simulink model "SWC_TCF"  (R2020a)
settings: Solver=FixedStepDiscrete  StartTime=0.0  StopTime=0.01  FixedStep=0.001  RelTol=1e-3
values from neighbouring files (symbols this model uses):
  CAL_TCF_AgTrqTubeCAy_af32 = 0.0    [SWC_TCF_DataDictionary.sldd]
  CAL_TCF_flgUsePlossCompa_b = 0.0    [SWC_TCF_DataDictionary.sldd]
  CAL_TCF_HiSpdDirStop_f32 = 0.0    [SWC_TCF_DataDictionary.sldd]
  CAL_TCF_HiTrqDirStop_f32 = 0.0    [SWC_TCF_DataDictionary.sldd]
  CAL_TCF_IsCutOffFrq_f32 = 0.0    [SWC_TCF_DataDictionary.sldd]
  CAL_TCF_IsPwrLosCAx_af32 = 0.0    [SWC_TCF_DataDictionary.sldd]
  CAL_TCF_LdSubLqCAzGen_af32 = 0.0    [SWC_TCF_DataDictionary.sldd]
  CAL_TCF_LdSubLqCAzMot_af32 = 0.0    [SWC_TCF_DataDictionary.sldd]
  CAL_TCF_LdSubLqIdCAx_af32 = 0.0    [SWC_TCF_DataDictionary.sldd]
  CAL_TCF_LdSubLqIqCAy_af32 = 0.0    [SWC_TCF_DataDictionary.sldd]
  CAL_TCF_LoSpdDirStop_f32 = 0.0    [SWC_TCF_DataDictionary.sldd]
  CAL_TCF_LoTrqDirStop_f32 = 0.0    [SWC_TCF_DataDictionary.sldd]
  CAL_TCF_MotorPole_u8 = 0.0    [SWC_TCF_DataDictionary.sldd]
  CAL_TCF_NPwrLosCAy_af32 = 0.0    [SWC_TCF_DataDictionary.sldd]
  CAL_TCF_Psi_f32 = 0.0    [SWC_TCF_DataDictionary.sldd]
  CAL_TCF_PwrCompaElectCAz_af32 = 0.0    [SWC_TCF_DataDictionary.sldd]
  CAL_TCF_PwrCompaIsCAy_af32 = 0.0    [SWC_TCF_DataDictionary.sldd]
  CAL_TCF_PwrCompaSpdCAx_af32 = 0.0    [SWC_TCF_DataDictionary.sldd]
  CAL_TCF_PwrInputCutOffFrq_f32 = 0.0    [SWC_TCF_DataDictionary.sldd]
  CAL_TCF_PwrLossCAz_af32 = 0.0    [SWC_TCF_DataDictionary.sldd]
  CAL_TCF_PwrTrqCalcSpdThrH_f32 = 0.0    [SWC_TCF_DataDictionary.sldd]
  CAL_TCF_PwrTrqCalcSpdThrL_f32 = 0.0    [SWC_TCF_DataDictionary.sldd]
  CAL_TCF_PwrTrqTubeCAy_af32 = 0.0    [SWC_TCF_DataDictionary.sldd]
  CAL_TCF_SpeedCtlMode_u8 = 0.0    [SWC_TCF_DataDictionary.sldd]
  CAL_TCF_TempStrMax_f32 = 0.0    [SWC_TCF_DataDictionary.sldd]
  CAL_TCF_TempStrMin_f32 = 0.0    [SWC_TCF_DataDictionary.sldd]
  CAL_TCF_TempStrPlossFact_f32 = 0.0    [SWC_TCF_DataDictionary.sldd]
  CAL_TCF_TrqCalcMonCountTrh_s16 = 0.0    [SWC_TCF_DataDictionary.sldd]
  CAL_TCF_TrqCalcMonDebTrh_s16 = 0.0    [SWC_TCF_DataDictionary.sldd]
  CAL_TCF_TrqCalcMonErrRst_b = 0.0    [SWC_TCF_DataDictionary.sldd]
  CAL_TCF_TrqMechCutOffFrq_f32 = 0.0    [SWC_TCF_DataDictionary.sldd]
  CAL_TCF_TrqTubeNCAx_af32 = 0.0    [SWC_TCF_DataDictionary.sldd]
  GLB_TCF_BwELect_u8 = 0.0    [SWC_TCF_DataDictionary.sldd]
  GLB_TCF_BwGene_u8 = 0.0    [SWC_TCF_DataDictionary.sldd]
  GLB_TCF_CircAge_f32 = 0.0    [SWC_TCF_DataDictionary.sldd]
  GLB_TCF_DigtValue_u16 = 0.0    [SWC_TCF_DataDictionary.sldd]
  GLB_TCF_FwELect_u8 = 0.0    [SWC_TCF_DataDictionary.sldd]
  GLB_TCF_FwGene_u8 = 0.0    [SWC_TCF_DataDictionary.sldd]
  GLB_TCF_MotorBw_u8 = 0.0    [SWC_TCF_DataDictionary.sldd]
  GLB_TCF_MotorFw_u8 = 0.0    [SWC_TCF_DataDictionary.sldd]
  GLB_TCF_MotorStop_u8 = 0.0    [SWC_TCF_DataDictionary.sldd]
  GLB_TCF_NegvTrq_u8 = 0.0    [SWC_TCF_DataDictionary.sldd]
  GLB_TCF_PosvTrq_u8 = 0.0    [SWC_TCF_DataDictionary.sldd]
  GLB_TCF_ZeroTrq_u8 = 0.0    [SWC_TCF_DataDictionary.sldd]
  PRV_CalFltFrq_1ms = 0.0    [SWC_TCF_DataDictionary.sldd]
  PRV_IsCalFltFrq_1ms = 0.0    [SWC_TCF_DataDictionary.sldd]
  Tbl_cos_table = 0.0    [SWC_TCF_DataDictionary.sldd]
  Tbl_sin_table = 0.0    [SWC_TCF_DataDictionary.sldd]
  TCF_PwrCompaGenCAz_af32 = 0.0    [SWC_TCF_DataDictionary.sldd]
undefined symbols (not defined in the file or in its folder): CAL_TOM_AgTrqFltTs_f32, CAL_TOM_PwrTrqFltTs_f32
libraries: simulink x9
(part 2 of 2)

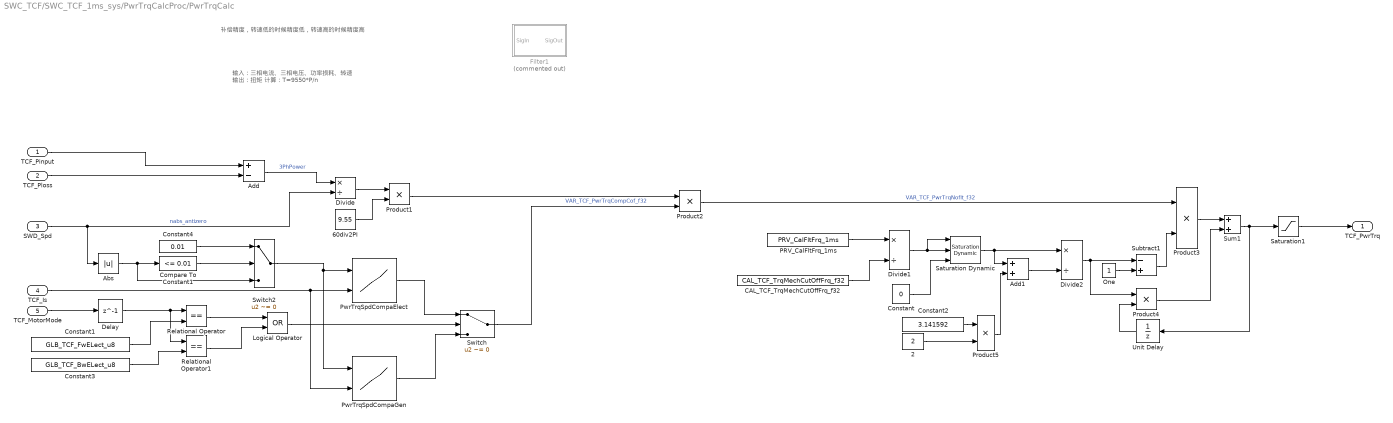
== system SWC_TCF/SWC_TCF_1ms_sys/PwrTrqCalcProc/PwrTrqCalc ==
  note: 补偿精度，转速低的时候精度低，转速高的时候精度高
  note: 输入：三相电流、三相电压、功率损耗、转速
      | 输出：扭矩
      | 计算：T=9550*P/n
  TCF_Pinput : Inport
  TCF_Ploss : Inport  Port=2
  SWD_Spd : Inport  Port=3
  TCF_Is : Inport  Port=4
  TCF_MotorMode : Inport  Port=5
  2 : Constant  Value=2  OutDataTypeStr=single
  60div2PI : Constant  Value=9.55  OutDataTypeStr=single
  Abs : Abs
  Add : Sum  Inputs=+-
  Add1 : Sum
  CAL_TCF_TrqMechCutOffFrq_f32 : Constant  Value=CAL_TCF_TrqMechCutOffFrq_f32
  Compare To Constant1 : simulink/Logic and Bit Operations/Compare To Constant  relop=<=  const=0.01  OutDataTypeStr=boolean
  Constant : Constant  Value=0  OutDataTypeStr=single
  Constant1 : Constant  Value=GLB_TCF_FwELect_u8  OutDataTypeStr=uint8
  Constant2 : Constant  Value=3.141592  OutDataTypeStr=single
  Constant3 : Constant  Value=GLB_TCF_BwELect_u8  OutDataTypeStr=uint8
  Constant4 : Constant  Value=0.01  OutDataTypeStr=single
  Delay : Delay  DelayLength=1  InitialCondition=0
  Divide : Product  Inputs=*/
  Divide1 : Product  Inputs=*/
  Divide2 : Product  Inputs=*/
  Filter1 : Subsystem  Commented=on
  Logical Operator : Logic  Operator=OR  AllPortsSameDT=off  OutDataTypeStr=boolean
  One : Constant  OutDataTypeStr=single
  PRV_CalFltFrq_1ms : Constant  Value=PRV_CalFltFrq_1ms
  Product{1..5} (5 alike) : Product
  PwrTrqSpdCompaElect : Lookup_n-D  BreakpointsForDimension1=CAL_TCF_PwrCompaSpdCAx_af32  BreakpointsForDimension2=CAL_TCF_PwrCompaIsCAy_af32  Table=CAL_TCF_PwrCompaElectCAz_af32  UseLastTableValue=on  InternalRulePriority=Speed  RndMeth=Simplest  InputSameDT=on
  PwrTrqSpdCompaGen : Lookup_n-D  BreakpointsForDimension1=CAL_TCF_PwrCompaSpdCAx_af32  BreakpointsForDimension2=CAL_TCF_PwrCompaIsCAy_af32  Table=TCF_PwrCompaGenCAz_af32  UseLastTableValue=on  InternalRulePriority=Speed  RndMeth=Simplest  InputSameDT=on
  Relational Operator : RelationalOperator  Operator===  OutDataTypeStr=boolean  RndMeth=Simplest
  Relational Operator1 : RelationalOperator  Operator===  OutDataTypeStr=boolean  RndMeth=Simplest
  Saturation Dynamic : simulink/Discontinuities/Saturation Dynamic  OutMin=[]  OutMax=[]  OutDataTypeStr=Inherit: Same as second input  OutDataType=fixdt(1, 16)  OutScaling=2^-10  DoSatur=off
  Saturation1 : Saturate  UpperLimit=500  LowerLimit=-500
  Subtract1 : Sum  Inputs=-+
  Sum1 : Sum
  Switch : Switch  Criteria=u2 ~= 0
  Switch2 : Switch  Criteria=u2 ~= 0
  Unit Delay : UnitDelay  SampleTime=-1  HasFrameUpgradeWarning=on
  TCF_PwrTrq : Outport  VectorParamsAs1DForOutWhenUnconnected=off
  wires:
  SWD_Spd/1 -> Abs/1, Divide/2  "nabs_antizero"
  60div2PI/1 -> Product1/2
  Divide/1 -> Product1/1
  Add/1 -> Divide/1  "3PhPower"
  TCF_Ploss/1 -> Add/2
  Product1/1 -> Product2/1
  TCF_Pinput/1 -> Add/1
  Sum1/1 -> Saturation1/1, Unit Delay/1
  Divide1/1 -> Saturation Dynamic/1, Saturation Dynamic/2
  Product5/1 -> Add1/2
  Product4/1 -> Sum1/2
  Unit Delay/1 -> Product4/2
  One/1 -> Subtract1/2
  Product2/1 -> Product3/1  "VAR_TCF_PwrTrqNoflt_f32"
  Add1/1 -> Divide2/2
  Divide2/1 -> Product4/1, Subtract1/1
  Constant/1 -> Saturation Dynamic/3
  Subtract1/1 -> Product3/2
  PRV_CalFltFrq_1ms/1 -> Divide1/1
  Saturation Dynamic/1 -> Divide2/1, Add1/1
  Product3/1 -> Sum1/1
  2/1 -> Product5/2
  Constant2/1 -> Product5/1
  CAL_TCF_TrqMechCutOffFrq_f32/1 -> Divide1/2
  Saturation1/1 -> TCF_PwrTrq/1
  Switch2/1 -> PwrTrqSpdCompaGen/1, PwrTrqSpdCompaElect/1
  TCF_Is/1 -> PwrTrqSpdCompaGen/2, PwrTrqSpdCompaElect/2
  PwrTrqSpdCompaElect/1 -> Switch/1
  PwrTrqSpdCompaGen/1 -> Switch/3
  TCF_MotorMode/1 -> Delay/1
  Constant3/1 -> Relational Operator1/2
  Relational Operator/1 -> Logical Operator/1
  Constant1/1 -> Relational Operator/2
  Relational Operator1/1 -> Logical Operator/2
  Logical Operator/1 -> Switch/2
  Switch/1 -> Product2/2  "VAR_TCF_PwrTrqCompCof_f32"
  Abs/1 -> Switch2/3, Compare To Constant1/1
  Constant4/1 -> Switch2/1
  Compare To Constant1/1 -> Switch2/2
  Delay/1 -> Relational Operator1/1, Relational Operator/1

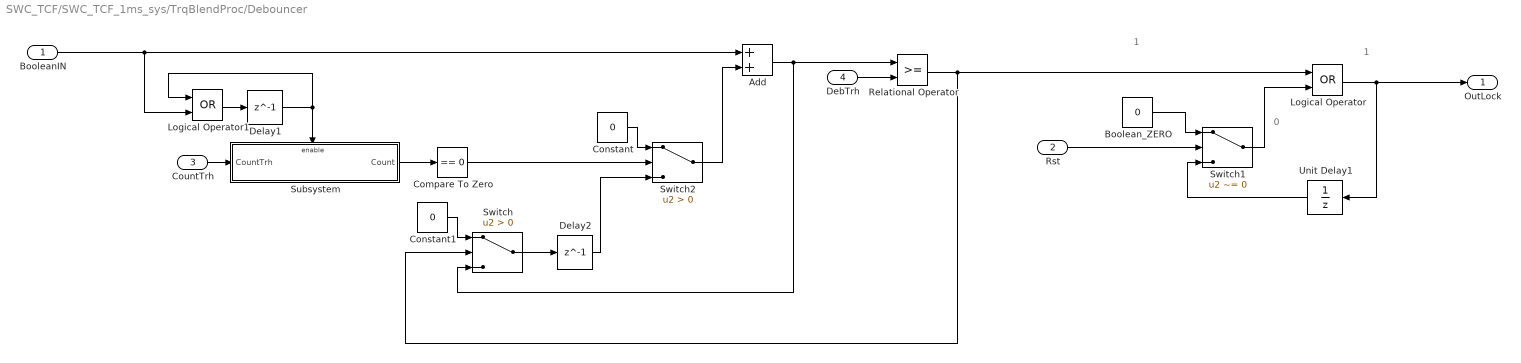
== system SWC_TCF/SWC_TCF_1ms_sys/TrqBlendProc/Debouncer ==
  note: 0
  note: 1
  note: 1
  BooleanIN : Inport
  Rst : Inport  Port=2
  CountTrh : Inport  Port=3
  DebTrh : Inport  Port=4
  Add : Sum
  Boolean_ZERO : Constant  Value=0  OutDataTypeStr=boolean
  Compare To Zero : simulink/Logic and Bit Operations/Compare To Zero  relop===  OutDataTypeStr=boolean
  Constant : Constant  Value=0  OutDataTypeStr=int16
  Constant1 : Constant  Value=0  OutDataTypeStr=int16
  Delay1 : Delay  DelayLength=1
  Delay2 : Delay  DelayLength=1
  Logical Operator : Logic  Operator=OR  AllPortsSameDT=off  OutDataTypeStr=boolean
  Logical Operator1 : Logic  Operator=OR  AllPortsSameDT=off  OutDataTypeStr=boolean
  Relational Operator : RelationalOperator  OutDataTypeStr=boolean  RndMeth=Simplest
  Subsystem : Subsystem
  Switch : Switch  Criteria=u2 > Threshold
  Switch1 : Switch  Criteria=u2 ~= 0
  Switch2 : Switch  Criteria=u2 > Threshold
  Unit Delay1 : UnitDelay  SampleTime=-1  HasFrameUpgradeWarning=on
  OutLock : Outport  VectorParamsAs1DForOutWhenUnconnected=off
  wires:
  Constant1/1 -> Switch/1
  Switch/1 -> Delay2/1
  DebTrh/1 -> Relational Operator/2
  Relational Operator/1 -> Logical Operator/1, Switch/2
  BooleanIN/1 -> Add/1, Logical Operator1/2
  Unit Delay1/1 -> Switch1/3
  Switch1/1 -> Logical Operator/2
  Rst/1 -> Switch1/2
  Boolean_ZERO/1 -> Switch1/1
  Logical Operator/1 -> Unit Delay1/1, OutLock/1
  Subsystem/1(Count) -> Compare To Zero/1
  Compare To Zero/1 -> Switch2/2
  Constant/1 -> Switch2/1
  Switch2/1 -> Add/2
  Delay1/1 -> Logical Operator1/1, Subsystem/Enable
  Logical Operator1/1 -> Delay1/1
  CountTrh/1 -> Subsystem/1(CountTrh)
  Add/1 -> Switch/3, Relational Operator/1
  Delay2/1 -> Switch2/3

== system SWC_TCF/SWC_TCF_1ms_sys/TrqBlendProc/TrqBlend ==
  TCF_PwrTrq_TubeH : Inport
  TCF_PwrTrq_TubeL : Inport  Port=2
  TCF_CurrAgTrq_TubeH : Inport  Port=3
  TCF_CurrAgTrq_TubeL : Inport  Port=4
  TubeSelector2 : Stateflow chart  TreatAsAtomicUnit=on
  TubeSelector3 : Stateflow chart  Commented=on  TreatAsAtomicUnit=on
  TCF_BlendTrq : Outport  VectorParamsAs1DForOutWhenUnconnected=off
  TCF_TrqCalcMonRslt : Outport  Port=2
  wires:
  TubeSelector2/2(TubeErr) -> TCF_TrqCalcMonRslt/1
  TubeSelector2/1(TubeOut) -> TCF_BlendTrq/1
  TCF_PwrTrq_TubeH/1 -> TubeSelector2/1(CH1H)
  TCF_PwrTrq_TubeL/1 -> TubeSelector2/2(CH1L)
  TCF_CurrAgTrq_TubeH/1 -> TubeSelector2/3(CH2H)
  TCF_CurrAgTrq_TubeL/1 -> TubeSelector2/4(CH2L)

== system SWC_TCF/SWC_TCF_1ms_sys/TrqBlendProc/TrqTube ==
  PwrTrqCalcEnable : Inport
  TCF_PwrTrq : Inport  Port=2
  SWD_Spd : Inport  Port=3
  TCF_CurrAgTrq : Inport  Port=4
  1-D Lookup Table : Lookup_n-D  NumberOfTableDimensions=1  BreakpointsForDimension1=CAL_TCF_TrqTubeNCAx_af32  Table=CAL_TCF_AgTrqTubeCAy_af32  InternalRulePriority=Speed  RndMeth=Simplest  InputSameDT=on
  Abs : Abs
  Add : Sum
  Add1 : Sum  Inputs=+-
  Add2 : Sum
  Add3 : Sum  Inputs=+-
  Cal_PowerTrqTube_T : Lookup_n-D  NumberOfTableDimensions=1  BreakpointsForDimension1=CAL_TCF_TrqTubeNCAx_af32  Table=CAL_TCF_PwrTrqTubeCAy_af32  InternalRulePriority=Speed  RndMeth=Simplest  InputSameDT=on
  Switch : Switch  Criteria=u2 > Threshold
  TCF_PwrTrq_TubeH : Outport  VectorParamsAs1DForOutWhenUnconnected=off
  TCF_PwrTrq_TubeL : Outport  Port=2  VectorParamsAs1DForOutWhenUnconnected=off
  TCF_CurrAgTrq_TubeH : Outport  Port=3  VectorParamsAs1DForOutWhenUnconnected=off
  TCF_CurrAgTrq_TubeL : Outport  Port=4  VectorParamsAs1DForOutWhenUnconnected=off
  wires:
  Add/1 -> TCF_PwrTrq_TubeH/1
  Add1/1 -> TCF_PwrTrq_TubeL/1
  Cal_PowerTrqTube_T/1 -> Add1/2, Add/2
  SWD_Spd/1 -> Abs/1
  1-D Lookup Table/1 -> Add3/2, Add2/2
  TCF_CurrAgTrq/1 -> Switch/3, Add3/1, Add2/1
  Add2/1 -> TCF_CurrAgTrq_TubeH/1
  Add3/1 -> TCF_CurrAgTrq_TubeL/1
  TCF_PwrTrq/1 -> Switch/1
  Switch/1 -> Add1/1, Add/1  "VAR_TCF_PwrTrqfltcomp_f32"
  Abs/1 -> 1-D Lookup Table/1, Cal_PowerTrqTube_T/1
  PwrTrqCalcEnable/1 -> Switch/2

== system SWC_TCF/SWC_TCF_1ms_sys/CurrAgTrqCalcProc/CurrAgTrqCalc/Filter1 ==
  note: 0.1
  SigIn : Inport
  Add : Sum  Inputs=-+
  Add1 : Sum
  CAL_TOM_AgTrqFltTs_f32 : Constant  Value=CAL_TOM_AgTrqFltTs_f32  OutDataTypeStr=single
  Constant1 : Constant  OutDataTypeStr=single
  Product : Product
  Product1 : Product
  Unit Delay : UnitDelay  SampleTime=-1  HasFrameUpgradeWarning=on
  SigOut : Outport  VectorParamsAs1DForOutWhenUnconnected=off
  wires:
  Add1/1 -> SigOut/1, Unit Delay/1
  CAL_TOM_AgTrqFltTs_f32/1 -> Add/1, Product/2
  Constant1/1 -> Add/2
  Unit Delay/1 -> Product1/2
  Add/1 -> Product1/1
  SigIn/1 -> Product/1
  Product1/1 -> Add1/2
  Product/1 -> Add1/1

== system SWC_TCF/SWC_TCF_1ms_sys/CurrAgTrqCalcProc/MotorModeJdg/MotorMode ==
  note: 前进、电动
  note: 后退发电
  note: 前进发电
  note: 后退电动
  note: 前进电动
  note: 前进、发电
  note: 后退、电动
  note: 后退、发电or停止
  note: 3
  note: 4
  note: 1
  note: 2
  TCF_TrqDir : Inport
  TCF_nDir : Inport  Port=2
  GLB_TOM_MotorBw_u8 : Constant  Value=GLB_TCF_MotorBw_u8
  GLB_TOM_MotorFw_u8 : Constant  Value=GLB_TCF_MotorFw_u8
  GLB_TOM_NegvTrq_u8 : Constant  Value=GLB_TCF_NegvTrq_u8
  GLB_TOM_PosvTrq_u8 : Constant  Value=GLB_TCF_PosvTrq_u8
  If : If  NumInputs=6  IfExpression=(u1==u3)&(u4==u5)  ElseIfExpressions=(u1==u2)&(u4==u6),(u1~=u3)&(u4~=u6)
  If Action Subsystem : Subsystem  TreatAsAtomicUnit=on
  If Action Subsystem1 : Subsystem  TreatAsAtomicUnit=on
  If Action Subsystem2 : Subsystem  TreatAsAtomicUnit=on
  If Action Subsystem3 : Subsystem  TreatAsAtomicUnit=on
  Merge : Merge  Inputs=4  InitialOutput=1
  TCF_MotorMod : Outport  VectorParamsAs1DForOutWhenUnconnected=off
  wires:
  Merge/1 -> TCF_MotorMod/1
  If Action Subsystem3/1(Out1) -> Merge/4
  If Action Subsystem2/1(Out1) -> Merge/2
  If Action Subsystem1/1(Out1) -> Merge/1
  If Action Subsystem/1(Out1) -> Merge/3
  If/4 -> If Action Subsystem3/Action
  If/3 -> If Action Subsystem/Action
  If/2 -> If Action Subsystem2/Action
  If/1 -> If Action Subsystem1/Action
  GLB_TOM_NegvTrq_u8/1 -> If/6
  GLB_TOM_PosvTrq_u8/1 -> If/5
  GLB_TOM_MotorBw_u8/1 -> If/3
  GLB_TOM_MotorFw_u8/1 -> If/2
  TCF_TrqDir/1 -> If/4
  TCF_nDir/1 -> If/1

== system SWC_TCF/SWC_TCF_1ms_sys/CurrAgTrqCalcProc/MotorModeJdg/TrqDir ==
  note: 2
  note: 1
  note: 0
  note: -3
  note: 3
  TCF_CurrAgTrqFlt : Inport
  CAL_TOM_HiTrqDirStop_f32 : Constant  Value=CAL_TCF_HiTrqDirStop_f32
  CAL_TOM_LoTrqDirStop_f32 : Constant  Value=CAL_TCF_LoTrqDirStop_f32
  GLB_TOM_NegvTrq_u8 : Constant  Value=GLB_TCF_NegvTrq_u8
  GLB_TOM_PosvTrq_u8 : Constant  Value=GLB_TCF_PosvTrq_u8
  GLB_TpcCod_ZeroTrq_u8 : Constant  Value=GLB_TCF_ZeroTrq_u8
  Logical Operator : Logic  AllPortsSameDT=off  OutDataTypeStr=boolean
  Relational Operator : RelationalOperator  OutDataTypeStr=boolean  RndMeth=Simplest
  Relational Operator1 : RelationalOperator  Operator=<=  OutDataTypeStr=boolean  RndMeth=Simplest
  Relational Operator2 : RelationalOperator  Operator=>  OutDataTypeStr=boolean  RndMeth=Simplest
  Switch : Switch  Criteria=u2 ~= 0
  Switch1 : Switch  Criteria=u2 ~= 0
  UnitDelay : UnitDelay  SampleTime=-1  HasFrameUpgradeWarning=on
  TCF_TrqDir : Outport  VectorParamsAs1DForOutWhenUnconnected=off
  wires:
  UnitDelay/1 -> Relational Operator/1, Relational Operator1/1, Relational Operator2/1
  GLB_TOM_NegvTrq_u8/1 -> Switch1/3
  GLB_TOM_PosvTrq_u8/1 -> Switch1/1
  Relational Operator2/1 -> Switch1/2
  Switch/1 -> TCF_TrqDir/1
  Switch1/1 -> Switch/3
  GLB_TpcCod_ZeroTrq_u8/1 -> Switch/1
  Logical Operator/1 -> Switch/2
  Relational Operator1/1 -> Logical Operator/2
  Relational Operator/1 -> Logical Operator/1
  TCF_CurrAgTrqFlt/1 -> UnitDelay/1
  CAL_TOM_LoTrqDirStop_f32/1 -> Relational Operator/2
  CAL_TOM_HiTrqDirStop_f32/1 -> Relational Operator2/2, Relational Operator1/2

== system SWC_TCF/SWC_TCF_1ms_sys/CurrAgTrqCalcProc/MotorModeJdg/nDir ==
  note: 10
  note: 2
  note: 1
  note: 0
  note: -10
  SWD_Spd : Inport
  CAL_TOM_HiSpdDirStop_f32 : Constant  Value=CAL_TCF_HiSpdDirStop_f32
  CAL_TOM_LoSpdDirStop_f32 : Constant  Value=CAL_TCF_LoSpdDirStop_f32
  GLB_TOM_MotorBw_u8 : Constant  Value=GLB_TCF_MotorBw_u8
  GLB_TOM_MotorFw_u8 : Constant  Value=GLB_TCF_MotorFw_u8
  GLB_TOM_MotorStop_u8 : Constant  Value=GLB_TCF_MotorStop_u8
  Logical Operator : Logic  AllPortsSameDT=off  OutDataTypeStr=boolean
  Relational Operator : RelationalOperator  OutDataTypeStr=boolean  RndMeth=Simplest
  Relational Operator1 : RelationalOperator  Operator=<=  OutDataTypeStr=boolean  RndMeth=Simplest
  Relational Operator2 : RelationalOperator  Operator=>  OutDataTypeStr=boolean  RndMeth=Simplest
  Switch : Switch  Criteria=u2 ~= 0
  Switch1 : Switch  Criteria=u2 ~= 0
  TCF_nDir : Outport  VectorParamsAs1DForOutWhenUnconnected=off
  wires:
  Switch1/1 -> Switch/3
  GLB_TOM_MotorBw_u8/1 -> Switch1/3
  GLB_TOM_MotorFw_u8/1 -> Switch1/1
  Relational Operator2/1 -> Switch1/2
  Switch/1 -> TCF_nDir/1
  GLB_TOM_MotorStop_u8/1 -> Switch/1
  SWD_Spd/1 -> Relational Operator/1, Relational Operator1/1, Relational Operator2/1
  CAL_TOM_LoSpdDirStop_f32/1 -> Relational Operator/2
  Logical Operator/1 -> Switch/2
  Relational Operator1/1 -> Logical Operator/2
  Relational Operator/1 -> Logical Operator/1
  CAL_TOM_HiSpdDirStop_f32/1 -> Relational Operator2/2, Relational Operator1/2

== system SWC_TCF/SWC_TCF_1ms_sys/PwrTrqCalcProc/PwrTrqCalc/Filter1 ==
  note: 0.1
  SigIn : Inport
  Add : Sum  Inputs=-+
  Add1 : Sum
  CAL_TOM_PwrTrqFltTs_f32 : Constant  Value=CAL_TOM_PwrTrqFltTs_f32  OutDataTypeStr=single
  Constant1 : Constant  OutDataTypeStr=single
  Product : Product
  Product1 : Product
  Unit Delay : UnitDelay  SampleTime=-1  HasFrameUpgradeWarning=on
  SigOut : Outport  VectorParamsAs1DForOutWhenUnconnected=off
  wires:
  Add1/1 -> SigOut/1, Unit Delay/1
  CAL_TOM_PwrTrqFltTs_f32/1 -> Add/1, Product/2
  Constant1/1 -> Add/2
  Unit Delay/1 -> Product1/2
  Add/1 -> Product1/1
  SigIn/1 -> Product/1
  Product1/1 -> Add1/2
  Product/1 -> Add1/1

== system SWC_TCF/SWC_TCF_1ms_sys/TrqBlendProc/Debouncer/Subsystem ==
  CountTrh : Inport
  Enable : EnablePort
  Add : Sum
  Constant : Constant  OutDataTypeStr=int16
  Constant1 : Constant  Value=0  OutDataTypeStr=int16
  Delay : Delay  DelayLength=1
  Relational Operator : RelationalOperator  OutDataTypeStr=boolean  RndMeth=Simplest
  Switch : Switch  Criteria=u2 > Threshold
  Count : Outport
  wires:
  Switch/1 -> Delay/1, Count/1
  Constant/1 -> Add/1
  Relational Operator/1 -> Switch/2
  Add/1 -> Relational Operator/1, Switch/3
  Constant1/1 -> Switch/1
  CountTrh/1 -> Relational Operator/2
  Delay/1 -> Add/2

== system SWC_TCF/SWC_TCF_1ms_sys/CurrAgTrqCalcProc/MotorModeJdg/MotorMode/If Action Subsystem ==
  Action Port : ActionPort  ActionPortLabel=elseif((u1~=u3)&(u4~=u6))
  GLB_TOM_FwELect_u8 : Constant  Value=GLB_TCF_FwELect_u8
  Out1 : Outport  VectorParamsAs1DForOutWhenUnconnected=off
  wires:
  GLB_TOM_FwELect_u8/1 -> Out1/1

== system SWC_TCF/SWC_TCF_1ms_sys/CurrAgTrqCalcProc/MotorModeJdg/MotorMode/If Action Subsystem1 ==
  Action Port : ActionPort  ActionPortLabel=if((u1==u3)&(u4==u5))
  GLB_TOM_BwELect_u8 : Constant  Value=GLB_TCF_BwELect_u8
  Out1 : Outport  VectorParamsAs1DForOutWhenUnconnected=off
  wires:
  GLB_TOM_BwELect_u8/1 -> Out1/1

== system SWC_TCF/SWC_TCF_1ms_sys/CurrAgTrqCalcProc/MotorModeJdg/MotorMode/If Action Subsystem2 ==
  Action Port : ActionPort  ActionPortLabel=elseif( (u1==u2)&(u4==u6))
  GLB_TOM_FwGene_u8 : Constant  Value=GLB_TCF_FwGene_u8
  Out1 : Outport  VectorParamsAs1DForOutWhenUnconnected=off
  wires:
  GLB_TOM_FwGene_u8/1 -> Out1/1

== system SWC_TCF/SWC_TCF_1ms_sys/CurrAgTrqCalcProc/MotorModeJdg/MotorMode/If Action Subsystem3 ==
  Action Port : ActionPort  ActionPortLabel=else
  GLB_TOM_BwGene_u8 : Constant  Value=GLB_TCF_BwGene_u8
  Out1 : Outport  VectorParamsAs1DForOutWhenUnconnected=off
  wires:
  GLB_TOM_BwGene_u8/1 -> Out1/1

== stateflow chart SWC_TCF/SWC_TCF_1ms_sys/TrqBlendProc/TrqBlend/TubeSelector2 ==
  settings: stateMachineType=MEALY_MACHINE
  note: 逻辑：两种扭矩计算方式相差很大则说明有问题
  note: 交叉，2在上
      | 包含，2在上
  note: 交叉，1在上
      | 包含，1在上
  note: 两通道完全分离
  (default) -> (junction 1)
  (junction 20) -> (junction 24) [order 2]
  (junction 1) -> (junction 20) [order 3]
  (junction 1) -> (junction 8) [order 2] : [CH2L>=CH1H]
  (junction 24) -> (junction 26)
  (junction 20) -> (junction 22) [order 1] : [CH1H>=CH2H]
  (junction 1) -> (junction 3) [order 1] : [CH1L>=CH2H]
  (junction 8) -> (junction 16) : {TubeOut=CAL_TCF_TrqInvalid_s16;}
  (junction 3) -> (junction 13) : {TubeOut=CAL_TCF_TrqInvalid_s16;}
  (junction 26) -> (junction 43) [order 2]
  (junction 22) -> (junction 32) [order 2]
  (junction 26) -> (junction 36) [order 1] : [CH2L>=CH1L]
  (junction 43) -> (junction 45) : {TubeOut=(CH1H+CH1L)/2;}
  (junction 22) -> (junction 28) [order 1] : [CH1L>=CH2L]
  (junction 32) -> (junction 34) : {TubeOut=(CH2H+CH2L)/2;}
  (junction 16) -> (junction 13)
  (junction 13) -> (junction 18) : {TubeErr=1;}
  (junction 36) -> (junction 38) : {TubeOut=(CH2L+CH1H)/2;}
  (junction 28) -> (junction 30) : {TubeOut=(CH1L+CH2H)/2;}
  (junction 45) -> (junction 38)
  (junction 34) -> (junction 30)
  (junction 38) -> (junction 48) : {TubeErr=0;}
  (junction 30) -> (junction 41) : {TubeErr=0;}
  data: TubeOut output single; TubeErr output boolean; CH1H input single; CH1L input single; CH2H input single; CH2L input single; CAL_TCF_TrqInvalid_s16 parameter int16

== stateflow chart SWC_TCF/SWC_TCF_1ms_sys/TrqBlendProc/TrqBlend/TubeSelector3 ==
  settings: stateMachineType=MEALY_MACHINE
  note: 逻辑：两种扭矩计算方式相差很大则说明有问题
  (default) -> (junction 1)
  (junction 20) -> (junction 24) [order 3]
  (junction 1) -> (junction 20) [order 3]
  (junction 1) -> (junction 3) [order 1] : [CH2H>=CH2L>=CH1H>=CH1L]
  (junction 1) -> (junction 8) [order 2] : [CH1H>=CH1L>=CH2H>=CH2L]
  (junction 20) -> (junction 22) [order 1] : [CH2H>=CH1H>=CH1L>=CH2L]
  (junction 20) -> (junction 32) [order 2] : [CH1H>=CH2H>=CH2L>=CH1L]
  (junction 24) -> (junction 43) [order 1] : [CH1H>=CH2H>=CH1L>=CH2L]
  (junction 24) -> (junction 36) [order 2] : [CH2H>=CH1H>=CH2L>=CH1L]
  (junction 36) -> (junction 38) : {TubeOut=(CH1H+CH2L)/2;}
  (junction 43) -> (junction 45) : {TubeOut=(CH2H+CH1L)/2;}
  (junction 22) -> (junction 30) : {TubeOut=(CH1H+CH1L)/2;}
  (junction 32) -> (junction 34) : {TubeOut=(CH2H+CH2L)/2;}
  (junction 3) -> (junction 13) : {TubeOut=CAL_TCF_TrqInvalid_s16;}
  (junction 8) -> (junction 16) : {TubeOut=CAL_TCF_TrqInvalid_s16;}
  (junction 16) -> (junction 13)
  (junction 13) -> (junction 18) : {TubeErr=1;}
  (junction 45) -> (junction 38)
  (junction 34) -> (junction 30)
  (junction 38) -> (junction 48) : {TubeErr=0;}
  (junction 30) -> (junction 41) : {TubeErr=0;}
  data: TubeOut output single; TubeErr output boolean; CH1H input single; CH1L input single; CH2H input single; CH2L input single; CAL_TCF_TrqInvalid_s16 parameter int16
